simulink model "LQR_Test"  (R2020a)
settings: Solver=VariableStepAuto  StartTime=0.0  StopTime=30  RelTol=1e-3
values from neighbouring files (symbols this model uses):
  body_rate_0 = [0;0;0]    [LQGControl.m]    (also in LQRControl.m; LQRcontrol_with_Integrator.m)
  Euler_0 = [0;0;0]    [LQGControl.m]    (also in LQRControl.m; LQRcontrol_with_Integrator.m)
  g = [0;0;9.8]    [LQGControl.m]    (also in LQRControl.m; LQRcontrol_with_Integrator.m)
  I = [[0.1,0,0];[0,0.1,0];[0,0,0.15]]    [LQGControl.m]    (also in LQRControl.m; LQRcontrol_with_Integrator.m)
  K = lqr(sys.A,sys.B,Q,R)    [LQGControl.m]    (also in LQRControl.m; LQRcontrol_with_Integrator.m; MPC.m = 0.028)
  m = 0.2    [LQGControl.m]    (also in LQRControl.m; LQRcontrol_with_Integrator.m; animation_LQG.m = transpose(m); animation_LQG_basic.m = transpose(m))
  NL = 1    [LQGControl.m]    (also in LQRControl.m = 0)
  Rn = 10    [Blocks_LQR.m]    (also in Blocks_LQRbasic.m = 0.01; LQGControl.m = 0.0001; LQRControl.m = 0.0001; LQRcontrol_with_Integrator.m)
  ts = 0.01    [LQGControl.m]    (also in LQRControl.m; LQRcontrol_with_Integrator.m)
  XYZ_0 = [0;0;0]    [LQGControl.m]    (also in LQRControl.m; LQRcontrol_with_Integrator.m)
undefined symbols (not defined in the file or in its folder): DiscIntNeverNeededParam, WindLevel
libraries: simulink x14
settings Model: NumberOfSteps=10  Creator=blaze8871  LastModifiedBy=Xrisostomos
settings DataIOCC: SaveTime=off

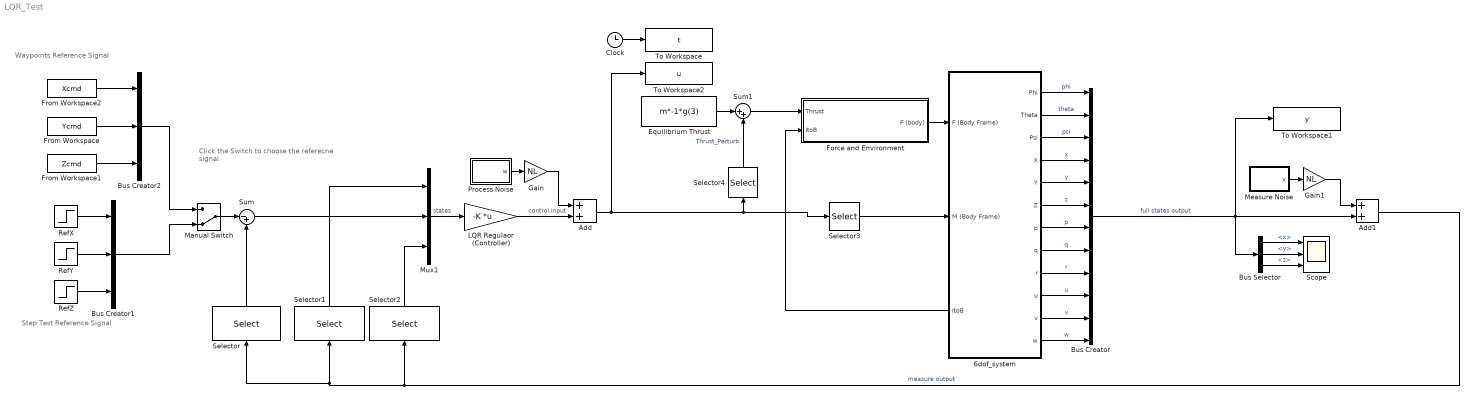
== system LQR_Test ==
  note: Click the Switch to choose the referecne signal
  note: Waypoints Reference Signal
  note: Step Test Reference Signal
  6dof_system : Subsystem
      settings: PortSchema="{\"entries\":[{\"content\":{\"sides\":[{\"content\":{\"connectorIds\":[\"In1\",\"In2\",\"Out13\"]},\"type\":\"ConnectorPlacement.EquallySpacedRectSide\",\"uuid\":\"a9788503-3606-44f5-8f01-204900b72727\"},{\"content\":{\"connectorIds\":[\"Out1\",\"Out2\",\"Out3\",\"Out4\",\"Out5\",\"Out6\",\"Out7\",\"Out8\",\"Out9\",\"Out10\",\"Out11\",\"Out12\"],\"side\":\"RIGHT\"},\"type\":\"ConnectorPlacement.EquallySpacedRectSide\",\"uuid\":\"4d9876d7-8651-4fde-9710-e2be9dd809ba\"},{\"content\":{\"connectorIds\":[],\"side\":\"TOP\"},\"type\":\"ConnectorPlacement.EquallySpacedRectSide\",\"uuid\":\"b5ce4f7f-c6d4-4ecb-8c48-bb3b2503bee9\"}]},\"type\":\"ConnectorPlacement.EquallySpacedConnector\",\"uuid\":\"5a2f747d-0d12-4160-9cbf-1dc51aae3069\"}],\"packageUris\":[\"http://schema.mathworks.com/mf0/Connector/19700101\"],\"version\":\"1.0\"}"
  Add : Sum
  Add1 : Sum
  Bus Creator : BusCreator  Inputs=12
  Bus Creator1 : BusCreator  Inputs=3
  Bus Creator2 : BusCreator  Inputs=3
  Bus Selector : BusSelector  OutputSignals=x,y,z
  Clock : Clock
  Equilibrium Thrust : Constant  Value=m*-1*g(3)
  Force and Environment : Subsystem
  From Workspace : FromWorkspace  VariableName=Ycmd  SampleTime=ts
  From Workspace1 : FromWorkspace  VariableName=Zcmd  SampleTime=ts
  From Workspace2 : FromWorkspace  VariableName=Xcmd  SampleTime=ts
  Gain : Gain  Gain=NL
  Gain1 : Gain  Gain=NL
  LQR Regulaor (Controller) : Gain  Gain=-K  Multiplication=Matrix(K*u)
  Manual Switch : ManualSwitch  CurrentSetting=0
  Measure Noise : Subsystem
  Mux1 : Mux  Inputs=3
  Process Noise : Subsystem
  RefX : Step  Time=3  SampleTime=0
  RefY : Step  Time=2  SampleTime=0
  RefZ : Step  SampleTime=0
  Scope : Scope  NumInputPorts=3
  Selector : Selector  InputPortWidth=12  IndexOptions=Index vector (dialog)  Indices=[4 5 6]  OutputSizes=1
  Selector1 : Selector  InputPortWidth=12  IndexOptions=Index vector (dialog)  Indices=[1 2 3]  OutputSizes=1
  Selector2 : Selector  InputPortWidth=12  IndexOptions=Index vector (dialog)  Indices=[7 8 9 10 11 12]  OutputSizes=1
  Selector3 : Selector  InputPortWidth=4  IndexOptions=Index vector (dialog)  Indices=[2 3 4]  OutputSizes=1
  Selector4 : Selector  InputPortWidth=4  IndexOptions=Index vector (dialog)  Indices=[1]  OutputSizes=1
  Sum : Sum  Inputs=|-+
  Sum1 : Sum  Inputs=|++
  To Workspace : ToWorkspace  VariableName=t  SampleTime=0.01
  To Workspace1 : ToWorkspace  VariableName=y  SampleTime=0.01
  To Workspace2 : ToWorkspace  VariableName=u  SampleTime=0.01
  wires:
  Force and Environment/1(F (body)) -> 6dof_system/1(F (Body Frame))
  6dof_system/13(ItoB) -> Force and Environment/2(ItoB)
  6dof_system/11(v) -> Bus Creator/11  "v"
  6dof_system/12(w) -> Bus Creator/12  "w"
  6dof_system/10(u) -> Bus Creator/10  "u"
  6dof_system/9(r) -> Bus Creator/9  "r"
  6dof_system/8(q) -> Bus Creator/8  "q"
  6dof_system/1(Phi) -> Bus Creator/1  "phi"
  6dof_system/2(Theta) -> Bus Creator/2  "theta"
  6dof_system/3(Psi) -> Bus Creator/3  "psi"
  6dof_system/4(X) -> Bus Creator/4  "x"
  6dof_system/5(Y) -> Bus Creator/5  "y"
  6dof_system/6(Z) -> Bus Creator/6  "z"
  6dof_system/7(p) -> Bus Creator/7  "p"
  Sum1/1 -> Force and Environment/1(Thrust)
  Bus Selector/1 -> Scope/1  "<x>"
  Bus Selector/2 -> Scope/2  "<y>"
  Bus Selector/3 -> Scope/3  "<z>"
  RefY/1 -> Bus Creator1/2
  RefZ/1 -> Bus Creator1/3
  RefX/1 -> Bus Creator1/1
  Selector/1 -> Sum/2
  Sum/1 -> Mux1/2
  Selector1/1 -> Mux1/1
  Selector2/1 -> Mux1/3
  Mux1/1 -> LQR Regulaor (Controller)/1  "states"
  Selector3/1 -> 6dof_system/2(M (Body Frame))
  Selector4/1 -> Sum1/2  "Thrust_Perturb"
  Equilibrium Thrust/1 -> Sum1/1
  From Workspace2/1 -> Bus Creator2/1
  From Workspace/1 -> Bus Creator2/2
  From Workspace1/1 -> Bus Creator2/3
  Manual Switch/1 -> Sum/1
  Bus Creator1/1 -> Manual Switch/2
  Bus Creator2/1 -> Manual Switch/1
  Process Noise/1(w) -> Gain/1
  Gain/1 -> Add/1
  LQR Regulaor (Controller)/1 -> Add/2  "control input"
  Gain1/1 -> Add1/1
  Bus Creator/1 -> Bus Selector/1, To Workspace1/1, Add1/2  "full states output"
  Measure Noise/1(v) -> Gain1/1
  Add1/1 -> Selector2/1, Selector/1, Selector1/1  "measure output"
  Clock/1 -> To Workspace/1
  Add/1 -> To Workspace2/1, Selector4/1, Selector3/1

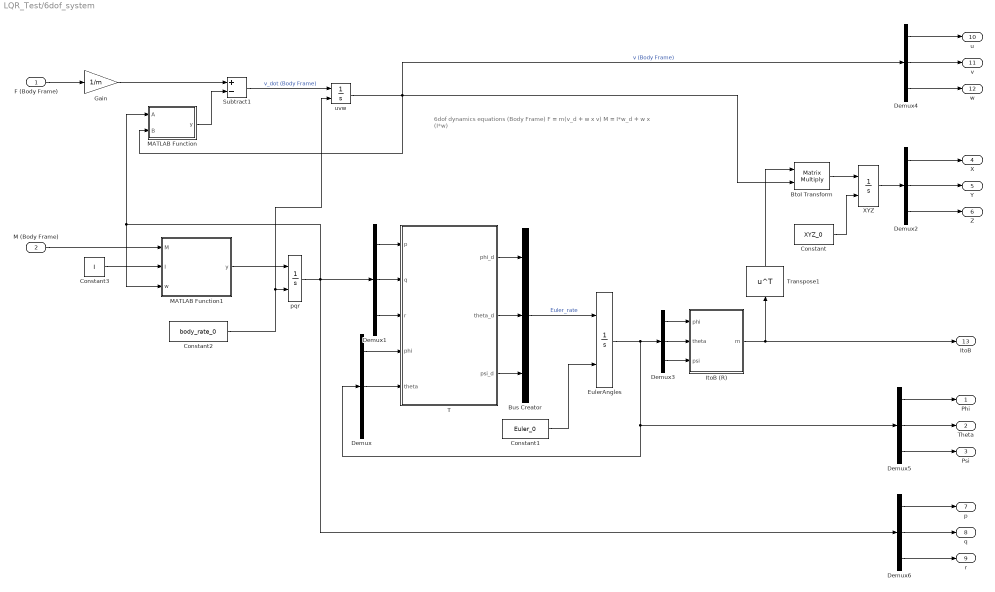
== system LQR_Test/6dof_system ==
  note: 6dof dynamics equations
      | (Body Frame)
      |
      | F = m(v_d + w x v)
      | M = I*w_d + w x (I*w)
  F (Body Frame) : Inport
  M (Body Frame) : Inport  Port=2
  BtoI Transform : Product  Multiplication=Matrix(*)
  Bus Creator : BusCreator  Inputs=3
  Constant : Constant  Value=XYZ_0  SampleTime=-1
  Constant1 : Constant  Value=Euler_0  SampleTime=-1
  Constant2 : Constant  Value=body_rate_0  SampleTime=-1
  Constant3 : Constant  Value=I
  Demux{,1..6} (7 alike) : Demux  Outputs=3
  EulerAngles : Integrator  InitialConditionSource=external  ContinuousStateAttributes='EulerAngle'
  Gain : Gain  Gain=1/m
  ItoB (R) : MATLAB Function  TreatAsAtomicUnit=on
  MATLAB Function : MATLAB Function  TreatAsAtomicUnit=on
  MATLAB Function1 : MATLAB Function  TreatAsAtomicUnit=on
  Subtract1 : Sum  Inputs=+-
  T : MATLAB Function  TreatAsAtomicUnit=on
  Transpose1 : Math  Operator=transpose  SaturateOnIntegerOverflow=on
  XYZ : Integrator  InitialConditionSource=external  ContinuousStateAttributes='XYZ'
  pqr : Integrator  InitialConditionSource=external  ContinuousStateAttributes='pqr'
  uvw : Integrator  InitialConditionSource=external  ContinuousStateAttributes='uvw'
  Phi : Outport
  Theta : Outport  Port=2
  Psi : Outport  Port=3
  X : Outport  Port=4
  Y : Outport  Port=5
  Z : Outport  Port=6
  p : Outport  Port=7
  q : Outport  Port=8
  r : Outport  Port=9
  u : Outport  Port=10
  v : Outport  Port=11
  w : Outport  Port=12
  ItoB : Outport  Port=13
  wires:
  F (Body Frame)/1 -> Gain/1
  T/1(phi_d) -> Bus Creator/1
  Bus Creator/1 -> EulerAngles/1  "Euler_rate"
  Demux3/2 -> ItoB (R)/2(theta)
  Demux/2 -> T/5(theta)
  Subtract1/1 -> uvw/1  "v_dot (Body Frame)"
  Demux1/1 -> T/1(p)
  T/2(theta_d) -> Bus Creator/2
  XYZ/1 -> Demux2/1
  Demux3/3 -> ItoB (R)/3(psi)
  T/3(psi_d) -> Bus Creator/3
  Gain/1 -> Subtract1/1
  Demux3/1 -> ItoB (R)/1(phi)
  Demux1/3 -> T/3(r)
  Demux/1 -> T/4(phi)
  uvw/1 -> Demux4/1, BtoI Transform/2, MATLAB Function/2(B)  "v (Body Frame)"
  Demux1/2 -> T/2(q)
  BtoI Transform/1 -> XYZ/1
  Constant1/1 -> EulerAngles/2
  Constant2/1 -> pqr/2, uvw/2
  Constant/1 -> XYZ/2
  Demux2/1 -> X/1
  Demux2/2 -> Y/1
  Demux2/3 -> Z/1
  Demux5/3 -> Psi/1
  Demux5/2 -> Theta/1
  Demux5/1 -> Phi/1
  EulerAngles/1 -> Demux3/1, Demux5/1, Demux/1
  MATLAB Function/1(y) -> Subtract1/2
  M (Body Frame)/1 -> MATLAB Function1/1(M)
  MATLAB Function1/1(y) -> pqr/1
  Constant3/1 -> MATLAB Function1/2(I)
  ItoB (R)/1(m) -> ItoB/1, Transpose1/1
  Transpose1/1 -> BtoI Transform/1
  Demux4/3 -> w/1
  Demux4/2 -> v/1
  Demux4/1 -> u/1
  pqr/1 -> Demux6/1, MATLAB Function1/3(w), MATLAB Function/1(A), Demux1/1
  Demux6/1 -> p/1
  Demux6/2 -> q/1
  Demux6/3 -> r/1

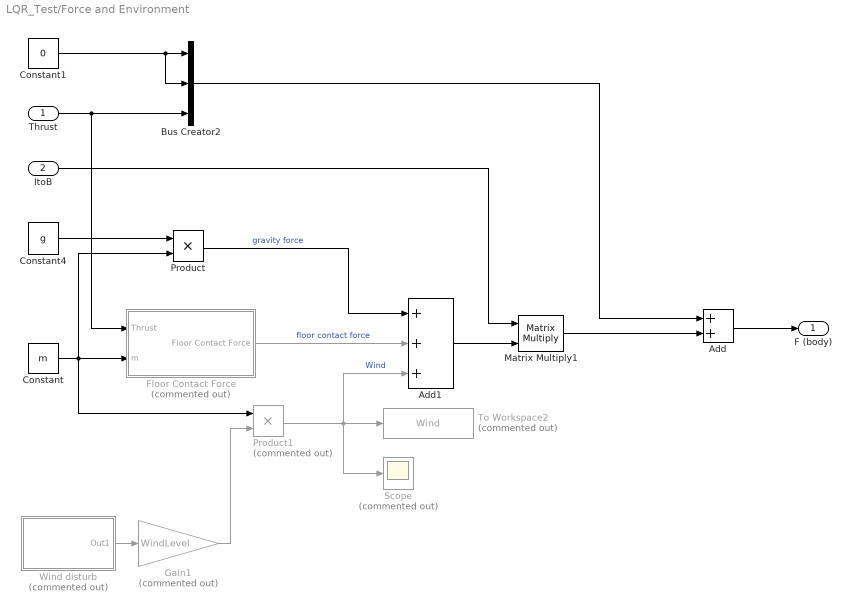
== system LQR_Test/Force and Environment ==
  Thrust : Inport
  ItoB : Inport  Port=2
  Add : Sum
  Add1 : Sum  Inputs=+++
  Bus Creator2 : BusCreator  Inputs=3
  Constant : Constant  Value=m  SampleTime=ts
  Constant1 : Constant  Value=0  SampleTime=-1
  Constant4 : Constant  Value=g  SampleTime=-1
  Floor Contact Force : Subsystem  Commented=on
  Gain1 : Gain  Commented=on  Gain=WindLevel
  Matrix Multiply1 : Product  Multiplication=Matrix(*)
  Product : Product
  Product1 : Product  Commented=on
  Scope : Scope  Commented=on
  To Workspace2 : ToWorkspace  Commented=on  VariableName=Wind  SampleTime=0.01
  Wind disturb : Subsystem  Commented=on
  F (body) : Outport
  wires:
  Wind disturb/1(Out1) -> Gain1/1
  Gain1/1 -> Product1/2
  Add/1 -> F (body)/1
  Thrust/1 -> Floor Contact Force/1(Thrust), Bus Creator2/3
  Constant4/1 -> Product/1
  Constant1/1 -> Bus Creator2/2, Bus Creator2/1
  Matrix Multiply1/1 -> Add/2
  Constant/1 -> Product/2, Floor Contact Force/2(m), Product1/1
  Bus Creator2/1 -> Add/1
  ItoB/1 -> Matrix Multiply1/1
  Product/1 -> Add1/1  "gravity force"
  Product1/1 -> Scope/1, To Workspace2/1, Add1/3  "Wind"
  Add1/1 -> Matrix Multiply1/2
  Floor Contact Force/1(Floor Contact Force) -> Add1/2  "floor contact force"

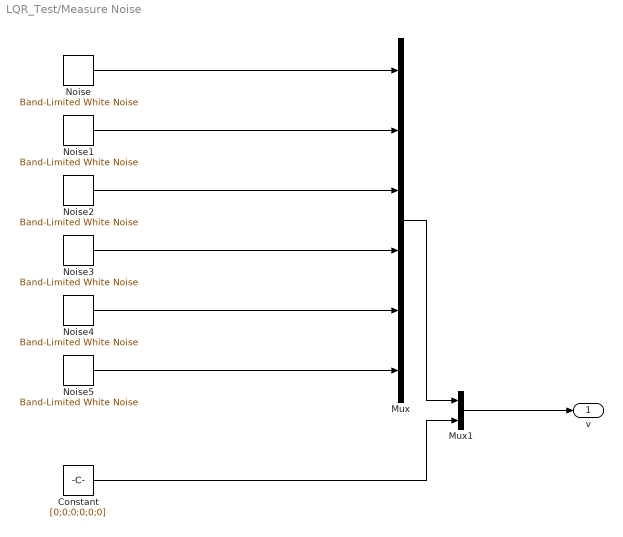
== system LQR_Test/Measure Noise ==
  " Noise" : simulink/Sources/Band-Limited White Noise  Cov=Rn*ts  Ts=ts  seed=[11432]
  " Noise1" : simulink/Sources/Band-Limited White Noise  Cov=Rn*ts  Ts=ts  seed=[13242]
  " Noise2" : simulink/Sources/Band-Limited White Noise  Cov=Rn*ts  Ts=ts  seed=[34124]
  " Noise3" : simulink/Sources/Band-Limited White Noise  Cov=Rn*ts  Ts=ts  seed=[41123]
  " Noise4" : simulink/Sources/Band-Limited White Noise  Cov=Rn*ts  Ts=ts  seed=[32144]
  " Noise5" : simulink/Sources/Band-Limited White Noise  Cov=Rn*ts  Ts=ts  seed=[14123]
  Constant : Constant  Value=[0;0;0;0;0;0]
  Mux : Mux  Inputs=6
  Mux1 : Mux  Inputs=2
  v : Outport
  wires:
  " Noise3"/1 -> Mux/4
  " Noise2"/1 -> Mux/3
  " Noise1"/1 -> Mux/2
  " Noise"/1 -> Mux/1
  " Noise4"/1 -> Mux/5
  " Noise5"/1 -> Mux/6
  Mux/1 -> Mux1/1
  Constant/1 -> Mux1/2
  Mux1/1 -> v/1

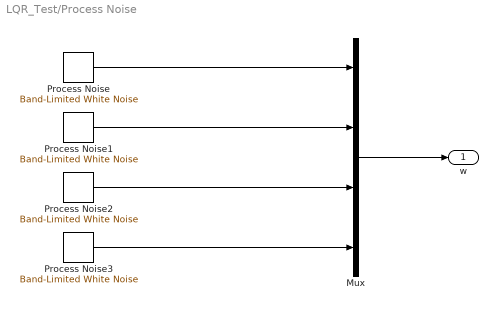
== system LQR_Test/Process Noise ==
  Mux : Mux
  Process Noise : simulink/Sources/Band-Limited White Noise  Cov=1e-3*ts  Ts=ts  seed=[11432]
  Process Noise1 : simulink/Sources/Band-Limited White Noise  Cov=1e-3*ts  Ts=ts  seed=[13242]
  Process Noise2 : simulink/Sources/Band-Limited White Noise  Cov=1e-3*ts  Ts=ts  seed=[34124]
  Process Noise3 : simulink/Sources/Band-Limited White Noise  Cov=1e-3*ts  Ts=ts  seed=[41123]
  w : Outport
  wires:
  Process Noise/1 -> Mux/1
  Mux/1 -> w/1
  Process Noise1/1 -> Mux/2
  Process Noise2/1 -> Mux/3
  Process Noise3/1 -> Mux/4

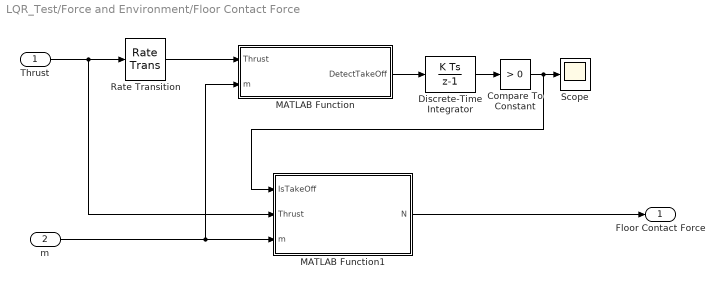
== system LQR_Test/Force and Environment/Floor Contact Force ==
  Thrust : Inport
  m : Inport  Port=2
  Compare To Constant : simulink/Logic and Bit Operations/Compare To Constant  relop=>  const=0  OutDataTypeStr=boolean
  Discrete-Time Integrator : DiscreteIntegrator  SampleTime=-1  LimitOutput=on  UpperSaturationLimit=1  ICPrevOutput=DiscIntNeverNeededParam  ICPrevScaledInput=DiscIntNeverNeededParam
  MATLAB Function : MATLAB Function  TreatAsAtomicUnit=on
  MATLAB Function1 : MATLAB Function  TreatAsAtomicUnit=on
  Rate Transition : RateTransition  OutPortSampleTime=ts
  Scope : Scope
  Floor Contact Force : Outport
  wires:
  Rate Transition/1 -> MATLAB Function/1(Thrust)
  Discrete-Time Integrator/1 -> Compare To Constant/1
  MATLAB Function/1(DetectTakeOff) -> Discrete-Time Integrator/1
  Compare To Constant/1 -> MATLAB Function1/1(IsTakeOff), Scope/1
  Thrust/1 -> MATLAB Function1/2(Thrust), Rate Transition/1
  m/1 -> MATLAB Function/2(m), MATLAB Function1/3(m)
  MATLAB Function1/1(N) -> Floor Contact Force/1

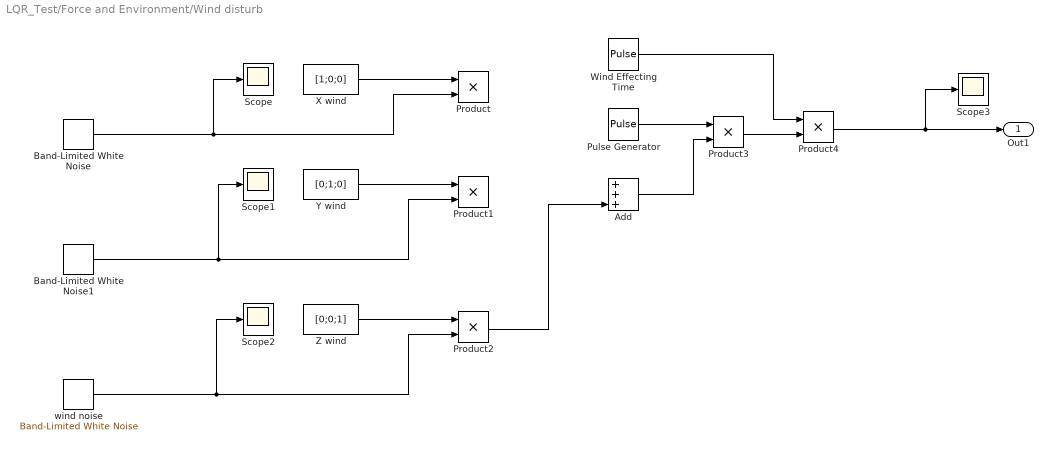
== system LQR_Test/Force and Environment/Wind disturb ==
  Add : Sum  Inputs=+++
  Band-Limited White Noise : simulink/Sources/Band-Limited White Noise  Cov=[0.1]  Ts=0.1  seed=[23341]
  Band-Limited White Noise1 : simulink/Sources/Band-Limited White Noise  Cov=[0.1]  Ts=0.1  seed=[41323]
  Product{,1..4} (5 alike) : Product
  Pulse Generator : DiscretePulseGenerator  PulseType=Time based  Period=2.5  PulseWidth=40
  Scope{,1..3} (4 alike) : Scope
  Wind Effecting Time : DiscretePulseGenerator  PulseType=Time based  Period=100  PulseWidth=10  PhaseDelay=3
  X wind : Constant  Value=[1;0;0]
  Y wind : Constant  Value=[0;1;0]
  Z wind : Constant  Value=[0;0;1]
  wind noise : simulink/Sources/Band-Limited White Noise  Cov=[1]  Ts=0.1  seed=[13244]
  Out1 : Outport
  wires:
  X wind/1 -> Product/1
  Band-Limited White Noise/1 -> Product/2, Scope/1
  Y wind/1 -> Product1/1
  Z wind/1 -> Product2/1
  Add/1 -> Product3/2
  Product2/1 -> Add/3
  Band-Limited White Noise1/1 -> Scope1/1, Product1/2
  wind noise/1 -> Scope2/1, Product2/2
  Pulse Generator/1 -> Product3/1
  Product3/1 -> Product4/2
  Wind Effecting Time/1 -> Product4/1
  Product4/1 -> Scope3/1, Out1/1

== matlab function LQR_Test/6dof_system/ItoB (R) ==
  data: phi input; m output; theta input; psi input
function m = fcn(phi,theta,psi)
    R_ItoV1= [[cos(psi) sin(psi) 0];[-sin(psi) cos(psi) 0];[0 0 1]];
    R_V1toV2 = [[cos(theta) 0 -sin(theta)];[0 1 0];[sin(theta) 0 cos(theta)]];
    R_V2toB = [[1 0 0];[0 cos(phi) sin(phi)];[0 -sin(phi) cos(phi)]];
    m = R_V2toB*R_V1toV2*R_ItoV1;

== matlab function LQR_Test/6dof_system/T ==
  data: p input; phi_d output; q input; r input; phi input; theta input; theta_d output; psi_d output
function [phi_d,theta_d,psi_d] = fcn(p,q,r,phi,theta)
    D = [[1 sin(phi)*tan(theta) cos(phi)*tan(theta)];
         [0 cos(phi) -sin(phi)];
         [0 sin(phi)/cos(theta) cos(phi)/cos(theta)]];
    euler_rate = D*[p;q;r]
    phi_d = euler_rate(1)
    theta_d = euler_rate(2)
    psi_d = euler_rate(3)

== matlab function LQR_Test/6dof_system/MATLAB Function ==
  data: A input; y output; B input
function y = fcn(A,B)
    y = cross(A,B);

== matlab function LQR_Test/6dof_system/MATLAB Function1 ==
  data: M input; y output; I input; w input
function y = fcn(M,I,w)
    y = inv(I)*(M-cross(w,I*w));

== matlab function LQR_Test/Force and Environment/Floor Contact Force/MATLAB Function ==
  data: Thrust input; DetectTakeOff output; m input
function DetectTakeOff = fcn(Thrust,m)
DetectTakeOff = 0;
if Thrust >= m*9.8
    DetectTakeOff = 1;
end

== matlab function LQR_Test/Force and Environment/Floor Contact Force/MATLAB Function1 ==
  data: IsTakeOff input; N output; Thrust input; m input
function N = fcn(IsTakeOff,Thrust,m)
if IsTakeOff == 0
    N = [0;0;m*9.8-Thrust];
else
    N = [0;0;0];
end
